simulink model "EPA_Walker"  (R2018a)
settings: Solver=FixedStepDiscrete  StartTime=0.0  StopTime=inf  FixedStep=0.001  RelTol=1e-3  EnableMultiTasking=on
model workspace (MAT data in the model file):
  MCOS : class17 (value not decoded)
undefined symbols (not defined in the file or in its folder): bits_current, bits_GRF, bits_Kd, bits_Kp, bits_position, bits_velocity, deadzone_in_TIB, deadzone_out_TIB, GRF_MAX, GRF_MIN, k_p_TIB, KD_MAX, KD_MIN, KP_MAX, KP_MIN, P_MAX, P_MIN, PressureFilter_CutOffFreq, PressureFilter_Gain, ReadingVoltage, T_MAX, T_MIN, V_MAX, V_MIN, voltageBias_GAS, voltageBias_GL, voltageBias_HAM, voltageBias_IL, voltageBias_POP, voltageBias_RF, voltageBias_SOL, voltageBias_TIB, voltageBias_VAS, voltageMultiplier_GAS, voltageMultiplier_GL, voltageMultiplier_HAM, voltageMultiplier_IL, voltageMultiplier_POP, voltageMultiplier_RF, voltageMultiplier_SOL, voltageMultiplier_TIB, voltageMultiplier_VAS, VoltageResolution
libraries: xpcethercatlib x139, simulink x19, peGeneralControl x18, slrtlib x9
(part 5 of 5)

== matlab function EPA_Walker/Ethernet Communication/Inputs/PAMs Right/MATLAB Function6 ==
  data: sensorValue input; pressure output; voltageMultiplier_HAM parameter; voltageBias_HAM parameter; ReadingVoltage parameter; VoltageResolution parameter
function pressure   = fcn(sensorValue,voltageMultiplier_HAM, voltageBias_HAM,ReadingVoltage, VoltageResolution)
pressure   = PressureSensor(sensorValue,voltageMultiplier_HAM, voltageBias_HAM,ReadingVoltage,VoltageResolution);
end

== matlab function EPA_Walker/Ethernet Communication/Inputs/PAMs Right/MATLAB Function7 ==
  data: sensorValue input; pressure output; voltageMultiplier_IL parameter; voltageBias_IL parameter; ReadingVoltage parameter; VoltageResolution parameter
function pressure   = fcn(sensorValue,voltageMultiplier_IL, voltageBias_IL,ReadingVoltage, VoltageResolution)
pressure   = PressureSensor(sensorValue,voltageMultiplier_IL, voltageBias_IL,ReadingVoltage,VoltageResolution);
end

== matlab function EPA_Walker/Ethernet Communication/Inputs/PAMs Right/MATLAB Function8 ==
  data: sensorValue input; pressure output; voltageMultiplier_GL parameter; voltageBias_GL parameter; ReadingVoltage parameter; VoltageResolution parameter
function pressure   = fcn(sensorValue,voltageMultiplier_GL, voltageBias_GL,ReadingVoltage, VoltageResolution)
pressure   = PressureSensor(sensorValue,voltageMultiplier_GL, voltageBias_GL,ReadingVoltage,VoltageResolution);
end

== matlab function EPA_Walker/Ethernet Communication/Outputs/Motor Right/Byte Splitting Position ==
  data: byte input; Pos_h output; Pos_l output
function [Pos_h,Pos_l] = fcn(byte)

Pos_l = bitand(byte,255);
Pos_h = bitshift(byte,-8);

== matlab function EPA_Walker/Ethernet Communication/Outputs/Motor Right/Byte Splitting Position1 ==
  data: byte input; Vel_h output; Vel_l output
function [Vel_h,Vel_l] = fcn(byte)

Vel_l = bitand(byte,15);
Vel_h = bitshift(byte,-4);

== matlab function EPA_Walker/Ethernet Communication/Outputs/Motor Right/Byte Splitting Position2 ==
  data: byte input; Kp_h output; Kp_l output
 function [Kp_h,Kp_l] = fcn(byte)

Kp_l = bitand(byte,255);
Kp_h = bitshift(byte,-8);

== matlab function EPA_Walker/Ethernet Communication/Outputs/Motor Right/Byte Splitting Position3 ==
  data: byte input; Kd_h output; Kd_l output
function [Kd_h,Kd_l] = fcn(byte)

Kd_l = bitand(byte,15);
Kd_h = bitshift(byte,-4);

== matlab function EPA_Walker/Ethernet Communication/Outputs/Motor Right/Byte Splitting Position4 ==
  data: byte input; Torque_h output; Torque_l output
function [Torque_h,Torque_l] = fcn(byte)

Torque_l = bitand(byte,255);
Torque_h = bitshift(byte,-8);

== matlab function EPA_Walker/Ethernet Communication/Outputs/Motor Right/Byte Splitting Position5 ==
  data: byte input; Pos_h output; Pos_l output
function [Pos_h,Pos_l] = fcn(byte)

Pos_l = bitand(byte,255);
Pos_h = bitshift(byte,-8);

== matlab function EPA_Walker/Ethernet Communication/Outputs/Motor Right/Byte Splitting Position6 ==
  data: byte input; Vel_h output; Vel_l output
function [Vel_h,Vel_l] = fcn(byte)

Vel_l = bitand(byte,15);
Vel_h = bitshift(byte,-4);

== matlab function EPA_Walker/Ethernet Communication/Outputs/Motor Right/Byte Splitting Position7 ==
  data: byte input; Kp_h output; Kp_l output
function [Kp_h,Kp_l] = fcn(byte)

Kp_l = bitand(byte,255);
Kp_h = bitshift(byte,-8);

== matlab function EPA_Walker/Ethernet Communication/Outputs/Motor Right/Byte Splitting Position8 ==
  data: byte input; Kd_h output; Kd_l output
function [Kd_h,Kd_l] = fcn(byte)

Kd_l = bitand(byte,15);
Kd_h = bitshift(byte,-4);

== matlab function EPA_Walker/Ethernet Communication/Outputs/Motor Right/Byte Splitting Position9 ==
  data: byte input; Torque_h output; Torque_l output
function [Torque_h,Torque_l] = fcn(byte)

Torque_l = bitand(byte,255);
Torque_h = bitshift(byte,-8);

== matlab function EPA_Walker/Ethernet Communication/Outputs/Motor Right/MATLAB Function ==
  data: x input; x_int output; P_MIN parameter; P_MAX parameter; bits_position parameter
function x_int = float_to_uint(x, P_MIN, P_MAX, bits_position)
    % Converts a float to an unsigned int, given range and number of bits_position %
    x_int = float_to_uint(x, P_MIN, P_MAX, bits_position);
end

== matlab function EPA_Walker/Ethernet Communication/Outputs/Motor Right/MATLAB Function1 ==
  data: x input; x_int output; V_MIN parameter; V_MAX parameter; bits_velocity parameter
function x_int = float_to_uint(x, V_MIN, V_MAX, bits_velocity)
    % Converts a float to an unsigned int, given range and number of bits_velocity %
    x_int = float_to_uint(x, V_MIN, V_MAX, bits_velocity);
end

== matlab function EPA_Walker/Ethernet Communication/Outputs/Motor Right/MATLAB Function2 ==
  data: x input; x_int output; KP_MIN parameter; KP_MAX parameter; bits_Kp parameter
function x_int = float_to_uint(x, KP_MIN, KP_MAX, bits_Kp)
    % Converts a float to an unsigned int, given range and number of bits_Kp %
    x_int = float_to_uint(x, KP_MIN, KP_MAX, bits_Kp);

end

== matlab function EPA_Walker/Ethernet Communication/Outputs/Motor Right/MATLAB Function3 ==
  data: x input; x_int output; KD_MIN parameter; KD_MAX parameter; bits_Kd parameter
function x_int = float_to_uint(x, KD_MIN, KD_MAX, bits_Kd)
    % Converts a float to an unsigned int, given range and number of bits_Kd %
    x_int = float_to_uint(x, KD_MIN, KD_MAX, bits_Kd);

end

== matlab function EPA_Walker/Ethernet Communication/Outputs/Motor Right/MATLAB Function4 ==
  data: x input; x_int output; T_MIN parameter; T_MAX parameter; bits_current parameter
function x_int = float_to_uint(x, T_MIN, T_MAX, bits_current)
    % Converts a float to an unsigned int, given range and number of bits_current %
    x_int = float_to_uint(x, T_MIN, T_MAX, bits_current);

end

== matlab function EPA_Walker/Ethernet Communication/Outputs/Motor Right/MATLAB Function5 ==
  data: x input; x_int output; P_MIN parameter; P_MAX parameter; bits_position parameter
function x_int = float_to_uint(x, P_MIN, P_MAX, bits_position)
    % Converts a float to an unsigned int, given range and number of bits_position %
    x_int = float_to_uint(x, P_MIN, P_MAX, bits_position);
end

== matlab function EPA_Walker/Ethernet Communication/Outputs/Motor Right/MATLAB Function6 ==
  data: x input; x_int output; V_MIN parameter; V_MAX parameter; bits_velocity parameter
function x_int = float_to_uint(x, V_MIN, V_MAX, bits_velocity)
    % Converts a float to an unsigned int, given range and number of bits_velocity %
    x_int = float_to_uint(x, V_MIN, V_MAX, bits_velocity);

end

== matlab function EPA_Walker/Ethernet Communication/Outputs/Motor Right/MATLAB Function7 ==
  data: x input; x_int output; KP_MIN parameter; KP_MAX parameter; bits_Kp parameter
function x_int = float_to_uint(x, KP_MIN, KP_MAX, bits_Kp)
    % Converts a float to an unsigned int, given range and number of bits_Kp %
    x_int = float_to_uint(x, KP_MIN, KP_MAX, bits_Kp);
end

== matlab function EPA_Walker/Ethernet Communication/Outputs/Motor Right/MATLAB Function8 ==
  data: x input; x_int output; KD_MIN parameter; KD_MAX parameter; bits_Kd parameter
function x_int = float_to_uint(x, KD_MIN, KD_MAX, bits_Kd)
    % Converts a float to an unsigned int, given range and number of bits_Kd %
    x_int = float_to_uint(x, KD_MIN, KD_MAX, bits_Kd);
end

== matlab function EPA_Walker/Ethernet Communication/Outputs/Motor Right/MATLAB Function9 ==
  data: x input; x_int output; T_MIN parameter; T_MAX parameter; bits_current parameter
function x_int = float_to_uint(x, T_MIN, T_MAX, bits_current)
    % Converts a float to an unsigned int, given range and number of bits_current %
    x_int = float_to_uint(x, T_MIN, T_MAX, bits_current);
end

== matlab function EPA_Walker/Motors/Motor Right/Motor Mode Handler ==
  data: Hip_Mode input; Hip_Mode_out output; Hip_position_des input; Hip_velocity_des input; Hip_Kp input; Hip_Kd input; Hip_Curret_des input; Hip_position_des_out output; Hip_velocity_des_out output; Hip_Kp_out output; Hip_Kd_out output; Hip_Curret_des_out output
function [Hip_Mode_out, Hip_position_des_out, Hip_velocity_des_out, Hip_Kp_out, Hip_Kd_out, Hip_Curret_des_out] = fcn(Hip_Mode, Hip_position_des, Hip_velocity_des, Hip_Kp, Hip_Kd, Hip_Curret_des)

[Hip_Mode_out, Hip_position_des_out, Hip_velocity_des_out, Hip_Kp_out, Hip_Kd_out, Hip_Curret_des_out] = Motor_handler(Hip_Mode, Hip_position_des, Hip_velocity_des, Hip_Kp, Hip_Kd, Hip_Curret_des);

end

== matlab function EPA_Walker/Motors/Motor Right/Motor Mode Handler1 ==
  data: Knee_Mode input; Knee_Mode_out output; Knee_position_des input; Knee_velocity_des input; Knee_Kp input; Knee_Kd input; Knee_Curret_des input; Knee_position_des_out output; Knee_velocity_des_out output; Knee_Kp_out output; Knee_Kd_out output; Knee_Curret_des_out output
function [Knee_Mode_out, Knee_position_des_out, Knee_velocity_des_out, Knee_Kp_out, Knee_Kd_out, Knee_Curret_des_out] = fcn(Knee_Mode, Knee_position_des, Knee_velocity_des, Knee_Kp, Knee_Kd, Knee_Curret_des)

[Knee_Mode_out, Knee_position_des_out, Knee_velocity_des_out, Knee_Kp_out, Knee_Kd_out, Knee_Curret_des_out] = Motor_handler(Knee_Mode, Knee_position_des, Knee_velocity_des, Knee_Kp, Knee_Kd, Knee_Curret_des);

end

== matlab function EPA_Walker/High Level Control/HL Right/Motor Modes ==
  data: isSwing input; Hip_mode output; Knee_mode output
function [Hip_mode, Knee_mode] = fcn(isSwing)

if isSwing == 1
    Hip_mode = 1;
    Knee_mode = 1;
elseif isSwing == 0
    Hip_mode = 2;
    Knee_mode = 2;
else
    Hip_mode = 0;
    Knee_mode = 0;
end
end

== matlab function EPA_Walker/PAMs/PAMs Right/GAS/Solenoids ==
  data: control input; intake output; inside_deadzone input; outtake output; inside_deadzone_1 output; deadzone_in input; deadzone_out input; PAMs_on input; System_on input; depressurize input
function [intake, outtake,inside_deadzone_1] = fcn(control, inside_deadzone, deadzone_in, deadzone_out,PAMs_on,System_on,depressurize)

[intake, outtake,inside_deadzone_1] = Solenoid(control, inside_deadzone, deadzone_in, deadzone_out,PAMs_on,System_on,depressurize);
    
  
end

== matlab function EPA_Walker/PAMs/PAMs Right/GL/Solenoids ==
  data: control input; intake output; inside_deadzone input; outtake output; inside_deadzone_1 output; deadzone_in input; deadzone_out input; PAMs_on input; System_on input; depressurize input
function [intake, outtake,inside_deadzone_1] = fcn(control, inside_deadzone, deadzone_in, deadzone_out,PAMs_on,System_on,depressurize)

[intake, outtake,inside_deadzone_1] = Solenoid(control, inside_deadzone, deadzone_in, deadzone_out,PAMs_on,System_on,depressurize);
    
  
end

== matlab function EPA_Walker/PAMs/PAMs Right/HAM/Solenoids ==
  data: control input; intake output; inside_deadzone input; outtake output; inside_deadzone_1 output; deadzone_in input; deadzone_out input; PAMs_on input; System_on input; depressurize input
function [intake, outtake,inside_deadzone_1] = fcn(control, inside_deadzone, deadzone_in, deadzone_out,PAMs_on,System_on,depressurize)

[intake, outtake,inside_deadzone_1] = Solenoid(control, inside_deadzone, deadzone_in, deadzone_out,PAMs_on,System_on,depressurize);
    
  
end

== matlab function EPA_Walker/PAMs/PAMs Right/IL/Solenoids ==
  data: control input; intake output; inside_deadzone input; outtake output; inside_deadzone_1 output; deadzone_in input; deadzone_out input; PAMs_on input; System_on input; depressurize input
function [intake, outtake,inside_deadzone_1] = fcn(control, inside_deadzone, deadzone_in, deadzone_out,PAMs_on,System_on,depressurize)

[intake, outtake,inside_deadzone_1] = Solenoid(control, inside_deadzone, deadzone_in, deadzone_out,PAMs_on,System_on,depressurize);
    
  
end

== matlab function EPA_Walker/PAMs/PAMs Right/POP/Solenoids ==
  data: control input; intake output; inside_deadzone input; outtake output; inside_deadzone_1 output; deadzone_in input; deadzone_out input; PAMs_on input; System_on input; depressurize input
function [intake, outtake,inside_deadzone_1] = fcn(control, inside_deadzone, deadzone_in, deadzone_out,PAMs_on,System_on,depressurize)

[intake, outtake,inside_deadzone_1] = Solenoid(control, inside_deadzone, deadzone_in, deadzone_out,PAMs_on,System_on,depressurize);
    
  
end

== matlab function EPA_Walker/PAMs/PAMs Right/RF/Solenoids ==
  data: control input; intake output; inside_deadzone input; outtake output; inside_deadzone_1 output; deadzone_in input; deadzone_out input; PAMs_on input; System_on input; depressurize input
function [intake, outtake,inside_deadzone_1] = fcn(control, inside_deadzone, deadzone_in, deadzone_out,PAMs_on,System_on,depressurize)

[intake, outtake,inside_deadzone_1] = Solenoid(control, inside_deadzone, deadzone_in, deadzone_out,PAMs_on,System_on,depressurize);
    
  
end

== matlab function EPA_Walker/PAMs/PAMs Right/SOL/Solenoids ==
  data: control input; intake output; inside_deadzone input; outtake output; inside_deadzone_1 output; deadzone_in input; deadzone_out input; PAMs_on input; System_on input; depressurize input
function [intake, outtake,inside_deadzone_1] = fcn(control, inside_deadzone, deadzone_in, deadzone_out,PAMs_on,System_on,depressurize)

[intake, outtake,inside_deadzone_1] = Solenoid(control, inside_deadzone, deadzone_in, deadzone_out,PAMs_on,System_on,depressurize);
    
  
end

== matlab function EPA_Walker/PAMs/PAMs Right/TIB/Solenoids ==
  data: control input; intake output; inside_deadzone input; outtake output; inside_deadzone_1 output; PAMs_on input; System_on input; deadzone_in_TIB parameter; deadzone_out_TIB parameter; depressurize input
function [intake, outtake,inside_deadzone_1] = fcn(control, inside_deadzone, PAMs_on,System_on, deadzone_in_TIB, deadzone_out_TIB, depressurize)

[intake, outtake,inside_deadzone_1] = Solenoid(control, inside_deadzone, deadzone_in_TIB, deadzone_out_TIB,PAMs_on,System_on,depressurize);
    
  
end

== matlab function EPA_Walker/PAMs/PAMs Right/VAS/Solenoids ==
  data: control input; intake output; inside_deadzone input; outtake output; inside_deadzone_1 output; deadzone_in input; deadzone_out input; PAMs_on input; System_on input; depressurize input
function [intake, outtake,inside_deadzone_1] = fcn(control, inside_deadzone, deadzone_in, deadzone_out,PAMs_on,System_on,depressurize)

[intake, outtake,inside_deadzone_1] = Solenoid(control, inside_deadzone, deadzone_in, deadzone_out,PAMs_on,System_on,depressurize);
    
  
end

== matlab function EPA_Walker/Safety /MATLAB Function1 ==
  data: Hip_motor_safe output; Knee_motor_safe output; Motors_safe output; flag output; Hip_Position input; Knee_Position input; flag_1 input
function [Hip_motor_safe, Knee_motor_safe,Motors_safe,flag]= fcn(Hip_Position, Knee_Position, flag_1)

flag = flag_1;
if flag == 0
    if Hip_Position >= -50 && Hip_Position <50
        Hip_motor_safe = 1;
    else
        Hip_motor_safe = 0;   
        flag = 1;
    end
    if Knee_Position >= -10 && Knee_Position <110
        Knee_motor_safe = 1;
    else
        Knee_motor_safe = 0;  
        flag = 1;
    end
    Motors_safe = double(Hip_motor_safe & Knee_motor_safe);
else
    if Hip_Position >= -50 && Hip_Position <50
        Hip_motor_safe = 1;
    else
        Hip_motor_safe = 0;   
        flag = 1;
    end

    if Knee_Position >= -5 && Knee_Position <110
        Knee_motor_safe = 1;
    else
        Knee_motor_safe = 0;  
        flag = 1;
    end
    Motors_safe = 0;
end

end
